simulink model "ModelF"  (R2018a)
settings: Solver=ode23tb  StartTime=0.0  StopTime=0.01  MaxStep=10e-6  RelTol=1e-3
undefined symbols (not defined in the file or in its folder): PWM12, PWM3
libraries: powerlib x19
settings Model: Creator=Simon  LastModifiedBy=Simon
settings SolverCC: InitialStep=10e-8

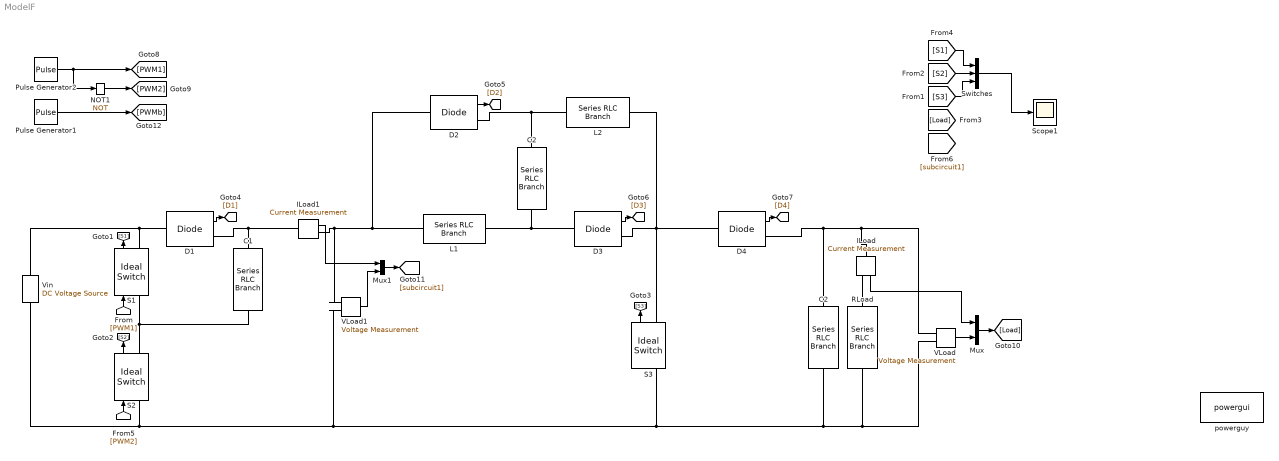
== system ModelF ==
  C1 : powerlib/Elements/Series RLC Branch  LConnTagsString=__new0  RConnTagsString=__new0  BranchType=C  Resistance=1  Inductance=1e-3  SetiL0=off  InitialCurrent=0  Capacitance=220e-5  Setx0=off  InitialVoltage=0  Measurements=None
  C2 : powerlib/Elements/Series RLC Branch  LConnTagsString=__new0  RConnTagsString=__new0  BranchType=C  Resistance=1  Inductance=1e-3  SetiL0=off  InitialCurrent=0  Capacitance=220e-5  Setx0=off  InitialVoltage=0  Measurements=None
  "C2 " : powerlib/Elements/Series RLC Branch  LConnTagsString=__new0  RConnTagsString=__new0  BranchType=C  Resistance=1  Inductance=1e-3  SetiL0=off  InitialCurrent=0  Capacitance=220e-5  Setx0=off  InitialVoltage=0  Measurements=None
  D{1..4} (4 alike) : powerlib/Power Electronics/Diode  Ron=0.001  Lon=0  Vf=0.8  IC=0  UseSnubber=0  Rs=500  Cs=250e-9  Measurements=on
  ILoad : powerlib/Measurements/Current Measurement  PhasorSimulation=off  OutputType=Complex  PSBequivalent=0
  ILoad1 : powerlib/Measurements/Current Measurement  PhasorSimulation=off  OutputType=Complex  PSBequivalent=0
  L1 : powerlib/Elements/Series RLC Branch  LConnTagsString=__new0  RConnTagsString=__new0  BranchType=L  Resistance=1  Inductance=150e-6  SetiL0=off  InitialCurrent=0  Capacitance=1e-6  Setx0=off  InitialVoltage=0  Measurements=None
  L2 : powerlib/Elements/Series RLC Branch  LConnTagsString=__new0  RConnTagsString=__new0  BranchType=L  Resistance=1  Inductance=150e-6  SetiL0=off  InitialCurrent=0  Capacitance=1e-6  Setx0=off  InitialVoltage=0  Measurements=None
  Mux : Mux  Inputs=2
  Mux1 : Mux  Inputs=2
  NOT1 : Logic  Operator=NOT  IconShape=distinctive  AllPortsSameDT=off  OutDataTypeStr=boolean
  Pulse Generator1 : DiscretePulseGenerator  PulseType=Time based  Period=1/50000  PulseWidth=PWM3  VectorParams1D=off
  Pulse Generator2 : DiscretePulseGenerator  PulseType=Time based  Period=1/50000  PulseWidth=PWM12  VectorParams1D=off
  RLoad : powerlib/Elements/Series RLC Branch  LConnTagsString=__new0  RConnTagsString=__new0  BranchType=R  Resistance=225  Inductance=1e-3  SetiL0=off  InitialCurrent=0  Capacitance=1e-6  Setx0=off  InitialVoltage=0  Measurements=None
  S1 : powerlib/Power Electronics/Ideal Switch  Ron=0.00001  Lon=0  IC=0  Rs=1e9  Cs=inf  Measurements=on
  S2 : powerlib/Power Electronics/Ideal Switch  Ron=0.00001  Lon=0  IC=0  Rs=1e9  Cs=inf  Measurements=on
  S3 : powerlib/Power Electronics/Ideal Switch  Ron=0.00001  Lon=0  IC=0  Rs=1e9  Cs=inf  Measurements=on
  Scope1 : Scope  NumInputPorts=3
  Switches : Mux  Inputs=3
  VLoad : powerlib/Measurements/Voltage Measurement  PhasorSimulation=off  OutputType=Complex  PSBequivalent=0
  VLoad1 : powerlib/Measurements/Voltage Measurement  PhasorSimulation=off  OutputType=Complex  PSBequivalent=0
  Vin : powerlib/Electrical Sources/DC Voltage Source  Amplitude=10  Measurements=None
  powerguy : powerlib/powergui  Priority=1  SimulationMode=Continuous  SampleTime=50e-6  frequency=60  Iterations=50  frequencyindice=0  Pbase=100e6  ErrMax=1e-4  UnitsV=kV  UnitsW=MW  buscounter=0  FunctionMessages=off  echomessages=off  EnableUseOfTLC=off  CurrentSourceSwitches=off  DisableSnubberDevices=off  DisableRonSwitches=off  DisableVfSwitches=off  DisplayEquations=off  SolverType=Tustin/Backward Euler (TBE)  Interpol=off  ExternalGateDelay=off  methode=off  Ts=100  x0status=blocks  SPID=on  SwTol=0  HookPort=off  RestoreLinks=warning  ResistiveCurrentMeasurement=off  Frange=[0:2:500]  Ylog=off  Xlog=on  ShowGrid=off  save=off  variable=ZData  structure=0  ZoomFFT=off  StartTime=0.0  cycles=1  DisplayStyle=1  fundamental=60  FreqAxis=off  MaxFrequency=1000  frequencyindicesteady=1  RmsSteady=1  display=off
  wires:
  Mux/1 -> [Load]
  ILoad/1 -> Mux/1
  VLoad/1 -> Mux/2
  S1/1 -> [S1]
  S2/1 -> [S2]
  S3/1 -> [S3]
  D1/1 -> [D1]
  D2/1 -> [D2]
  D3/1 -> [D3]
  D4/1 -> [D4]
  [S1] -> Switches/1
  [S2] -> Switches/2
  [S3] -> Switches/3
  Switches/1 -> Scope1/2
  [PWM1] -> S1/1
  [PWM2] -> S2/1
  Mux1/1 -> [subcircuit1]
  ILoad1/1 -> Mux1/1
  VLoad1/1 -> Mux1/2
  NOT1/1 -> [PWM2]
  Pulse Generator2/1 -> [PWM1], NOT1/1
  Pulse Generator1/1 -> [PWMb]
  connections:
  Vin/RConn1 -- D1/LConn1 -- S1/RConn1
  S1/LConn1 -- S2/RConn1 -- C1/RConn1
  L1/RConn1 -- D3/LConn1 -- C2/RConn1
  S2/LConn1 -- Vin/LConn1 -- VLoad1/LConn2 -- "C2 "/RConn1 -- VLoad/LConn2 -- RLoad/RConn1 -- S3/LConn1
  VLoad/LConn1 -- "C2 "/LConn1 -- D4/RConn1 -- ILoad/LConn1
  D1/RConn1 -- ILoad1/LConn1 -- C1/LConn1
  C2/LConn1 -- L2/LConn1 -- D2/RConn1
  RLoad/LConn1 -- ILoad/RConn1
  D3/RConn1 -- D4/LConn1 -- L2/RConn1 -- S3/RConn1
  D2/LConn1 -- ILoad1/RConn1 -- VLoad1/LConn1 -- L1/LConn1
